simulink model "mysvm_pdpwm"  (R2017b)
settings: Solver=ode45  StartTime=0.0  StopTime=0.02  RelTol=1e-3  EnableMultiTasking=on
values from neighbouring files (symbols this model uses):
  N = nlcinput(4) - 1    [MLNLC_m.m]    (also in MLPDPWM_m.m = pdpwminput(4) - 1; MLSVC_m.m = svcinput(4) - 1; MLSVM_m_HD.m = svminput(5) - 1; PlotSpaceVector.m = block.DialogPrm(1).Data - 1)
undefined symbols (not defined in the file or in its folder): f, m
libraries: powerlib x5, powerlib_meascontrol x4
settings Model: Creator=吴鸿达  LastModifiedBy=AdamWu
settings DataIOCC: LimitDataPoints=on  SaveFormat=Array
settings OptimizationCC: LifeSpan=inf
settings DebuggingCC: SolverPrmCheckMsg=warning  SFUnexpectedBacktrackingDiag=warning  SFNoUnconditionalDefaultTransitionDiag=warning  SFExecutionAtInitializationDiag=none
settings HardwareCC: ProdBitPerPointer=32  ProdBitPerSizeT=32  ProdBitPerPtrDiffT=32  ProdLargestAtomicFloat=None  ProdIntDivRoundTo=Undefined  ProdEndianess=Unspecified  ProdWordSize=32  ProdHWDeviceType=32-bit Generic
settings ModelReferenceCC: PropagateSignalLabelsOutOfModel=off
settings CodeAppCC: StateflowObjectComments=on
settings GRTTargetCC: TargetLangStandard=C89/C90 (ANSI)  GeneratePreprocessorConditionals=Disable all
settings ConfigComp: CovMetricSettings=dw  CovHtmlReporting=on  CovSaveCumulativeToWorkspaceVar=on  CovSaveSingleToWorkspaceVar=on  CovExternalEMLEnable=off  CovSFcnEnable=off
settings SimscapeCC: SimscapeNormalizeSystem=off

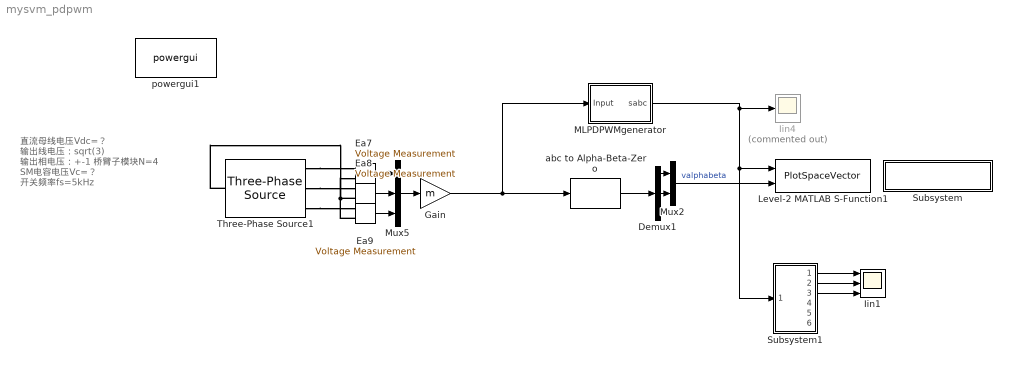
== system mysvm_pdpwm ==
  note: 直流母线电压Vdc=？
      |
      | 输出线电压：sqrt(3)
      | 输出相电压：+-1
      | 桥臂子模块N=4
      | SM电容电压Vc=？
      | 开关频率fs=5kHz
  Demux1 : Demux  Outputs=3
  Ea7 : powerlib/Measurements/Voltage Measurement  PhasorSimulation=off  OutputType=Complex  PSBequivalent=0
  Ea8 : powerlib/Measurements/Voltage Measurement  PhasorSimulation=off  OutputType=Complex  PSBequivalent=0
  Ea9 : powerlib/Measurements/Voltage Measurement  PhasorSimulation=off  OutputType=Complex  PSBequivalent=0
  Gain : Gain  Gain=m
  Iin1 : Scope  NumInputPorts=3
  Iin4 : Scope  Commented=on
  Level-2 MATLAB S-Function1 : M-S-Function  FunctionName=PlotSpaceVector  Parameters=level, vdc, rate, normalized, plot, hexagon, sw, disabled  mask{disabled=on, level=N, rate=200, vdc=2/50, normalized=on, plot=2, hexagon=off, sw=off}
      mask prompts: disabled "Disable Plot"; level "Voltage Level"; rate "Plot Rate"; vdc "DC Link Voltage"; plot "Plot Number"; sw "Show Switching"
  MLPDPWMgenerator : Subsystem  mask{level=N, fs=f, method=PDPWM}
      mask prompts: level "Voltage Level"; fs "Switching Frequency"; method "Methods"
      mask TypeOptions method: PDPWM | PODPWM | APODPWM
  Mux2 : Mux  Inputs=2
  Mux5 : Mux  Inputs=3
  Subsystem : Subsystem  mask{filename=SVPWM_sFunction.m}
      settings: AttributesFormatString=\n  OpenFcn=open('F:\研究生\matlab\PlotSpaceVector.m')
      mask Display:
      | patch([0 1 1 0], [0 0 1 1],[0.2 0.6 0.9])
      | disp('plotspacevector.m')
  Subsystem1 : Subsystem  mask{N=N}
      mask prompts: N "Voltage Level"
  Three-Phase Source1 : powerlib/Electrical Sources/Three-Phase Source  InternalConnection=Yn  VoltagePhases=off  Voltage=1.224745  PhaseAngle=0  Voltage_phases=[25e3 25e3 25e3]/sqrt(3)  PhaseAngles_phases=[0 -120 +120]  Frequency=50  NonIdealSource=off  SpecifyImpedance=off  Resistance=0.8929  Inductance=1e-3  ShortCircuitLevel=100e6  BaseVoltage=25e3  XRratio=7  BusType=swing  Pref=10e3  Qref=0  Prefabc=[10e3, 10e3, 10e3]  Qrefabc=[0, 0, 0]  Qmin=-inf  Qmax=inf
  abc to Alpha-Beta-Zero : powerlib_meascontrol/Transformations/abc to Alpha-Beta-Zero
      settings: SourceProductName=Simscape Power Systems
  powergui1 : powerlib/powergui  Priority=1  SimulationMode=Discrete  SampleTime=1e-6  frequency=60  Iterations=50  frequencyindice=50  Pbase=100e6  ErrMax=1e-4  UnitsV=kV  UnitsW=MW  buscounter=0  FunctionMessages=off  echomessages=off  EnableUseOfTLC=off  CurrentSourceSwitches=off  DisableSnubberDevices=off  DisableRonSwitches=off  DisableVfSwitches=off  DisplayEquations=off  SolverType=Tustin/Backward Euler (TBE)  Interpol=off  ExternalGateDelay=off  methode=off  Ts=100  x0status=blocks  SPID=on  SwTol=0  HookPort=off  RestoreLinks=warning  ResistiveCurrentMeasurement=off  Frange=[0:2:500]  Ylog=off  Xlog=on  ShowGrid=off  save=off  variable=ZData  structure=output  ZoomFFT=off  StartTime=0.0005  cycles=1  DisplayStyle=1  fundamental=50  FreqAxis=on  MaxFrequency=15000  frequencyindicesteady=1  RmsSteady=1  display=off
  wires:
  Ea9/1 -> Mux5/3
  Ea7/1 -> Mux5/1
  Ea8/1 -> Mux5/2
  abc to Alpha-Beta-Zero/1 -> Demux1/1
  Demux1/1 -> Mux2/1
  Demux1/2 -> Mux2/2
  Mux5/1 -> Gain/1
  Mux2/1 -> Level-2 MATLAB S-Function1/2  "valphabeta"
  Subsystem1/2(ab/bc/ca) -> Iin1/2
  Subsystem1/3(com) -> Iin1/3
  Subsystem1/1(abc) -> Iin1/1
  MLPDPWMgenerator/1(sabc) -> Iin4/1, Level-2 MATLAB S-Function1/1, Subsystem1/1("abc ")
  Gain/1 -> MLPDPWMgenerator/1(Input), abc to Alpha-Beta-Zero/1
  connections:
  Ea9/LConn2 -- Three-Phase Source1/LConn1 -- Ea7/LConn2 -- Ea8/LConn2
  Three-Phase Source1/RConn1 -- Ea7/LConn1
  Three-Phase Source1/RConn2 -- Ea8/LConn1
  Three-Phase Source1/RConn3 -- Ea9/LConn1

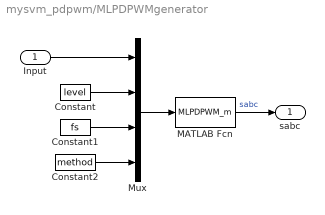
== system mysvm_pdpwm/MLPDPWMgenerator ==
  Input : Inport
  Constant : Constant  Value=level
  Constant1 : Constant  Value=fs
  Constant2 : Constant  Value=method
  MATLAB Fcn : MATLABFcn  MATLABFcn=MLPDPWM_m  OutputSignalType=real
  Mux : Mux
  sabc : Outport
  wires:
  MATLAB Fcn/1 -> sabc/1  "sabc"
  Input/1 -> Mux/1
  Constant1/1 -> Mux/3
  Constant/1 -> Mux/2
  Mux/1 -> MATLAB Fcn/1
  Constant2/1 -> Mux/4

== system mysvm_pdpwm/Subsystem ==

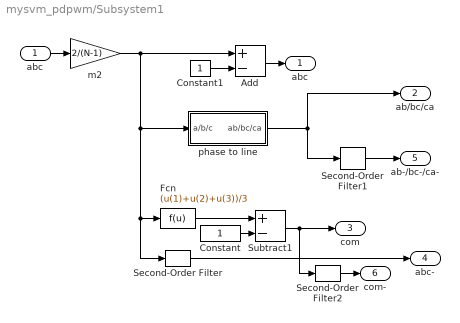
== system mysvm_pdpwm/Subsystem1 ==
  "abc " : Inport
  Add : Sum  Inputs=+-
  Constant : Constant
  Constant1 : Constant
  Fcn : Fcn  Expr=(u(1)+u(2)+u(3))/3
  Second-Order Filter : powerlib_meascontrol/Filters/Second-Order Filter  FilterType=Lowpass  Fo=1000  Zeta=0.707  Ts=0  Initialize=on  Vac_Init="[0,  0,  50]"  Vdc_Init=0  PlotResponse=off  FreqRange=[0, 500, 1]
      settings: SourceProductName=Simscape Power Systems  SourceProductBaseCode=PS
  Second-Order Filter1 : powerlib_meascontrol/Filters/Second-Order Filter  FilterType=Lowpass  Fo=1000  Zeta=0.707  Ts=0  Initialize=on  Vac_Init="[0,  0,  50]"  Vdc_Init=0  PlotResponse=off  FreqRange=[0, 500, 1]
      settings: SourceProductName=Simscape Power Systems  SourceProductBaseCode=PS
  Second-Order Filter2 : powerlib_meascontrol/Filters/Second-Order Filter  FilterType=Lowpass  Fo=1000  Zeta=0.707  Ts=0  Initialize=on  Vac_Init="[0,  0,  50]"  Vdc_Init=0  PlotResponse=off  FreqRange=[0, 500, 1]
      settings: SourceProductName=Simscape Power Systems  SourceProductBaseCode=PS
  Subtract1 : Sum  Inputs=+-
  m2 : Gain  Gain=2/(N-1)
  phase to line : Subsystem
  abc : Outport
  ab/bc/ca : Outport  Port=2
  com : Outport  Port=3
  abc- : Outport  Port=4
  ab-/bc-/ca- : Outport  Port=5
  com- : Outport  Port=6
  wires:
  Second-Order Filter/1 -> abc-/1
  Second-Order Filter2/1 -> com-/1
  Subtract1/1 -> com/1, Second-Order Filter2/1
  "abc "/1 -> m2/1
  Second-Order Filter1/1 -> ab-/bc-/ca-/1
  Fcn/1 -> Subtract1/1
  Constant/1 -> Subtract1/2
  m2/1 -> Add/1, phase to line/1(a/b/c), Second-Order Filter/1, Fcn/1
  Constant1/1 -> Add/2
  Add/1 -> abc/1
  phase to line/1(ab/bc/ca) -> Second-Order Filter1/1, ab/bc/ca/1

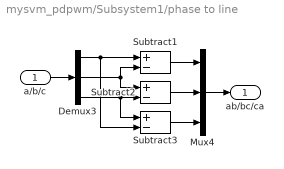
== system mysvm_pdpwm/Subsystem1/phase to line ==
  a/b/c : Inport
  Demux3 : Demux  Outputs=3
  Mux4 : Mux  Inputs=3
  Subtract1 : Sum  Inputs=+-
  Subtract2 : Sum  Inputs=+-
  Subtract3 : Sum  Inputs=+-
  ab/bc/ca : Outport
  wires:
  Subtract2/1 -> Mux4/2
  Subtract1/1 -> Mux4/1
  Demux3/2 -> Subtract2/1, Subtract1/2
  a/b/c/1 -> Demux3/1
  Mux4/1 -> ab/bc/ca/1
  Demux3/3 -> Subtract2/2, Subtract3/1
  Subtract3/1 -> Mux4/3
  Demux3/1 -> Subtract1/1, Subtract3/2
